simulink model "Maths_Pendulum"  (R2020a)
settings: Solver=VariableStepAuto  StartTime=0.0  StopTime=10  MaxStep=0.01  RelTol=1e-3
libraries: simulink_extras x1, simulink x1
settings Model: EnablePacing=on  Creator=Gleb  LastModifiedBy=Gleb

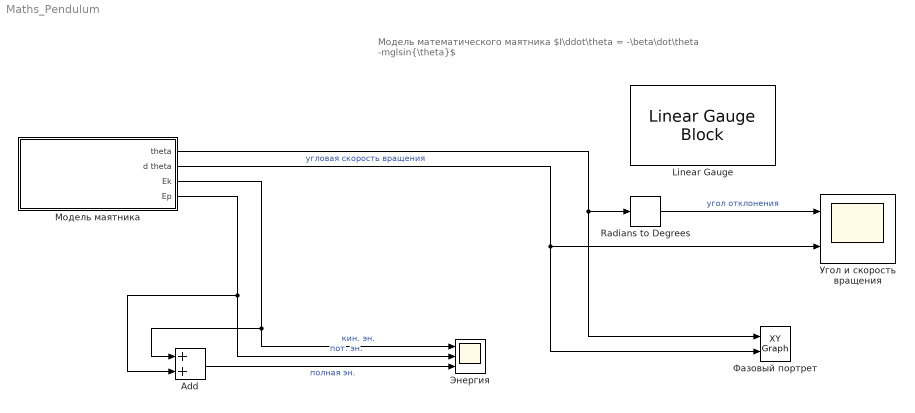
== system Maths_Pendulum ==
  note: Модель математического маятника
      | $I\ddot\theta = -\beta\dot\theta -mglsin{\theta}$
  Add : Sum
  Linear Gauge : LinearGaugeBlock  ScaleMin=-90  ScaleMax=90
  Radians to Degrees : simulink_extras/Transformations/Radians to Degrees
  Модель маятника : Subsystem  mask{m=1, l=1, g=9.8, startDegree=30, b=0.1}
      mask prompts: m "Масса"; l "Длина нити"; g "Ускорение своб. падения"; startDegree "Стартовый угол, градусы"; b "Коэффициент сопротивления"
      mask init:
      | I = m* l^2
  Угол и скорость вращения : Scope  NumInputPorts=2
  Фазовый портрет : simulink/Sinks/XY Graph  xmin=-10  xmax=10  ymin=-10  ymax=10  st=-1
  Энергия : Scope  NumInputPorts=3
  wires:
  Radians to Degrees/1 -> Угол и скорость вращения/1  "угол отклонения"
  Модель маятника/1(theta) -> Фазовый портрет/1, Radians to Degrees/1
  Модель маятника/2(d theta) -> Фазовый портрет/2, Угол и скорость вращения/2  "угловая скорость вращения"
  Модель маятника/3(Ek) -> Add/1, Энергия/1  "кин. эн."
  Модель маятника/4(Ep) -> Add/2, Энергия/2  "пот. эн."
  Add/1 -> Энергия/3  "полная эн."

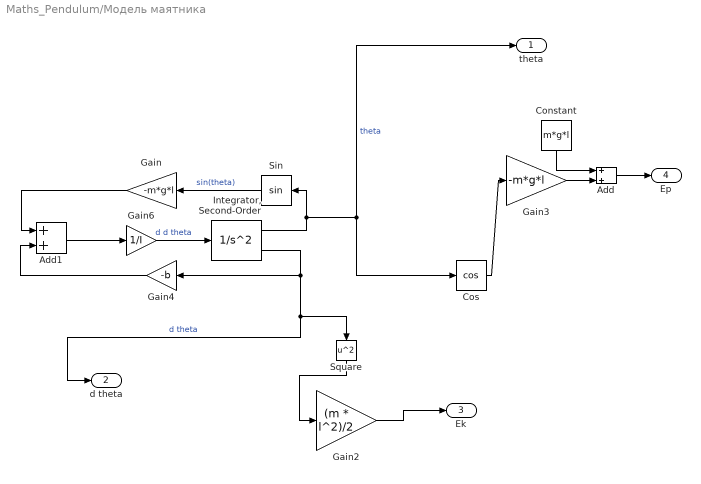
== system Maths_Pendulum/Модель маятника ==
  Add : Sum
  Add1 : Sum
  Constant : Constant  Value=m*g*l
  Cos : Trigonometry  Operator=cos
  Gain : Gain  Gain=-m*g*l
  Gain2 : Gain  Gain=(m * l^2)/2
  Gain3 : Gain  Gain=-m*g*l
  Gain4 : Gain  Gain=-b
  Gain6 : Gain  Gain=1/I
  "Integrator, Second-Order" : SecondOrderIntegrator  ICX=deg2rad(startDegree)
  Sin : Trigonometry
  Square : Math  Operator=square  SaturateOnIntegerOverflow=on
  theta : Outport
  d theta : Outport  Port=2
  Ek : Outport  Port=3
  Ep : Outport  Port=4
  wires:
  "Integrator, Second-Order"/1 -> theta/1, Cos/1, Sin/1  "theta"
  "Integrator, Second-Order"/2 -> Square/1, d theta/1, Gain4/1  "d theta"
  Sin/1 -> Gain/1  "sin(theta)"
  Gain/1 -> Add1/1
  Square/1 -> Gain2/1
  Gain2/1 -> Ek/1
  Cos/1 -> Gain3/1
  Constant/1 -> Add/1
  Gain3/1 -> Add/2
  Add/1 -> Ep/1
  Gain4/1 -> Add1/2
  Gain6/1 -> "Integrator, Second-Order"/1  "d d theta"
  Add1/1 -> Gain6/1
